simulink model "Super6"  (Simulink 5.0)
settings: Solver=ode45  StartTime=0.0  StopTime=10.0  RelTol=1e-3
settings Model: Creator=scaife  LastModifiedBy=scaife  ExtModeAutoUpdateStatusClock=off

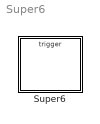
== system Super6 ==
  Super6 : Stateflow chart

== stateflow chart Super6 ==
  state A
    state A1
      state A1a
        state A1ai
        (default) -> A1ai
      (default) -> A1a
    (default) -> A1
  state B
    state B1
      state B1a
        state B1ai
        (default) -> B1ai
      (default) -> B1a
    (default) -> B1
  (default) -> A
  A -> B : E
  B -> A : E
  A1 -> B1 : F
  B1 -> A1 : F
  A1a -> B1a : G
  B1a -> A1a : G
  A1ai -> B1ai : H
  B1ai -> A1ai : H
  events: E input EITHER_EDGE_EVENT; G input EITHER_EDGE_EVENT; F input EITHER_EDGE_EVENT; H input EITHER_EDGE_EVENT
